simulink model "Model_4"  (R2020b)
settings: Solver=VariableStepAuto  StartTime=0.0  StopTime=10.0  RelTol=1e-3
settings Model: Creator=Akarsh  LastModifiedBy=Akarsh

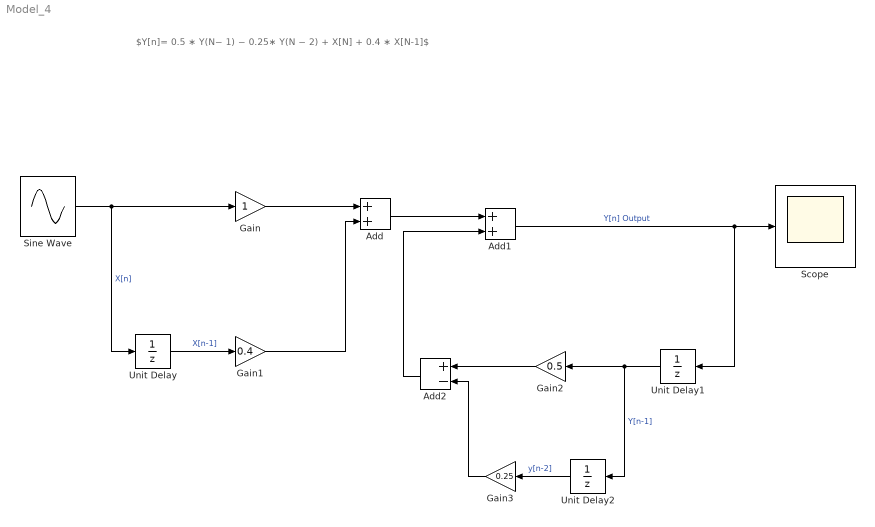
== system Model_4 ==
  note: $Y[n]= 0.5 ∗ Y(N− 1) − 0.25∗ Y(N − 2) + X[N] + 0.4 ∗ X[N-1]$
  Add : Sum
  Add1 : Sum
  Add2 : Sum  Inputs=+-
  Gain : Gain
  Gain1 : Gain  Gain=0.4
  Gain2 : Gain  Gain=0.5
  Gain3 : Gain  Gain=0.25
  Scope : Scope
  Sine Wave : Sin  SampleTime=0
  Unit Delay : UnitDelay  SampleTime=-1  HasFrameUpgradeWarning=on
  Unit Delay1 : UnitDelay  SampleTime=-1  HasFrameUpgradeWarning=on
  Unit Delay2 : UnitDelay  SampleTime=-1  HasFrameUpgradeWarning=on
  wires:
  Sine Wave/1 -> Gain/1, Unit Delay/1  "X[n]"
  Gain/1 -> Add/1
  Add/1 -> Add1/1
  Unit Delay/1 -> Gain1/1  "X[n-1]"
  Gain1/1 -> Add/2
  Add1/1 -> Scope/1, Unit Delay1/1  "Y[n] Output"
  Unit Delay1/1 -> Unit Delay2/1, Gain2/1  "Y[n-1]"
  Gain2/1 -> Add2/1
  Add2/1 -> Add1/2
  Unit Delay2/1 -> Gain3/1  "y[n-2]"
  Gain3/1 -> Add2/2
